simulink model "pos_edge_trig"  (Simulink 7.7)
settings: Solver=ode45  StartTime=0.0  StopTime=10.0  RelTol=1e-3
libraries: xbsIndex_r4 x3
settings Model: Creator=Lerwys  LastModifiedBy=Lerwys

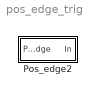
== system pos_edge_trig ==
  Pos_edge2 : Subsystem

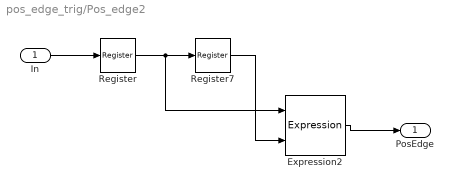
== system pos_edge_trig/Pos_edge2 ==
  In : Inport
  Expression2 : xbsIndex_r4/Expression  expression=a & ~b  align_bp=on  en=off  latency=0  precision=Full  arith_type=Unsigned  n_bits=16  bin_pt=0  dbl_ovrd=off  block_type=expr
  Register : xbsIndex_r4/Register  init=0  rst=off  en=off  dbl_ovrd=off  block_type=register
  Register7 : xbsIndex_r4/Register  init=0  rst=off  en=off  dbl_ovrd=off  block_type=register
  PosEdge : Outport
  wires:
  Register/1 -> Register7/1, Expression2/1
  Register7/1 -> Expression2/2
  In/1 -> Register/1
  Expression2/1 -> PosEdge/1
